simulink model "aie_hls"  (R2025a)
settings: Solver=VariableStepAuto  StartTime=0.0  StopTime=500  RelTol=1e-3
InitFcn:
  | %xmcCheckSlxPath(bdroot);
  | input = readcomplexdata('./sw/input.h');
undefined symbols (not defined in the file): S, Symmetric, vsva2197, xcvc1902
libraries: aieUtilities x2, aieDSP x1, aieBasic x1, hlsBasic x1, simulink x1, vmcUtilities x1, dspsrcs4 x1
settings Model: Creator=abehbood  LastModifiedBy=robg
settings SolverCC: AlgebraicLoopSolver=TrustRegion
settings DebuggingCC: UnconnectedInputMsg=warning  UnconnectedOutputMsg=warning  UnconnectedLineMsg=warning
settings ModelReferenceCC: EnableRefExpFcnMdlSchedulingChecks=on
settings SFSimCC: CustomCodeUndefinedFunction=UseInterfaceOnly
settings RTWCC: GPUComputeCapability=3.5  DLArmComputeVersion=19.05

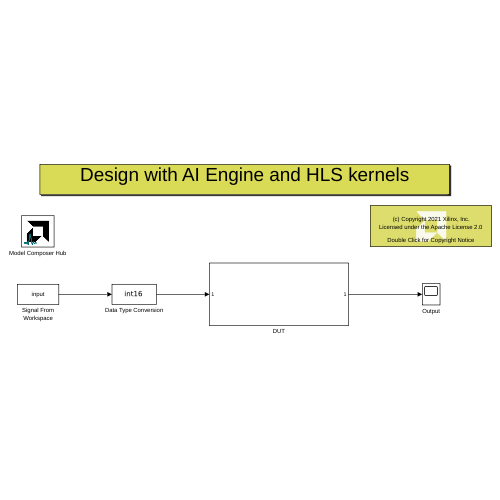
[thumbnail: Simulink's stored preview of the top-level diagram]
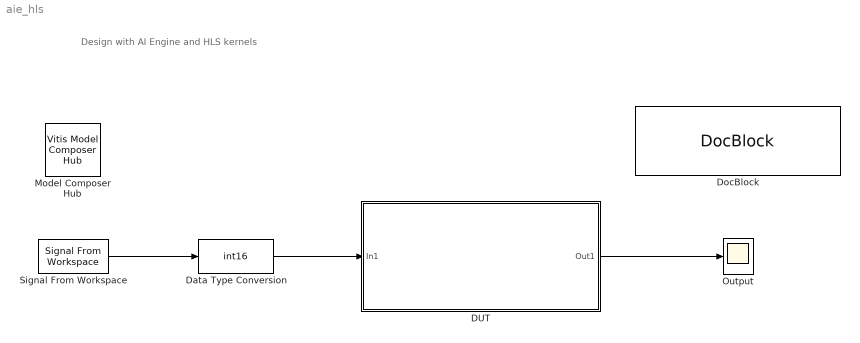
== system aie_hls ==
  note: Design with AI Engine and HLS kernels
  DUT : Subsystem
  Data Type Conversion : DataTypeConversion  OutDataTypeStr=int16  SaturateOnIntegerOverflow=off  RndMeth=Floor
  DocBlock : simulink/Model-Wide Utilities/DocBlock  DocumentType=Text  mask(DocBlock){}
      content=|
      | ///////////////////////////////////////////////////////////////////////////
      | // Copyright 2021 Xilinx
      | //
      | // Licensed under the Apache License, Version 2.0 (the "License");
      | // you may not use this file except in compliance with the License.
      | // You may obtain a copy of the License at
      | //
      | // http://www.apache.org/licenses/LICENSE-2.0
      | //
      | // Unless required by applicable law or agreed to in writing, software
      | // distributed under the License is distributed on an "AS IS" BASIS,
      | // WITHOUT WARRANTIES OR CONDITIONS OF ANY KIND, either express or implied.
      | // See the License for the specific language governing permissions and
      | // limitations under the License.
      | ///////////////////////////////////////////////////////////////////////////
      mask Display:
      | xmcDrawBlockIcon();
      | disp(['{\fontsize{10pt}(c) Copyright 2021' ' Xilinx, Inc.}\newline \newline '],'texmode','on');
      | disp('{\fontsize{10pt}Licensed under the Apache License 2.0}','texmode','on');
      | disp('\newline \newline \newline{\fontsize{10pt}Double Click for Copyright Notice}','texmode','on');
  Model Composer Hub : vmcUtilities/Vitis Model Composer Hub  Tag=genX  CodeGeneration=off  SubsystemName=DUT  BlockHierPath=aie_hls/DUT  CompilationType=VitisCompilation  SubsystemType=DUTNode  AIEArrayConfig=Use entire AIE array  StartColumn=1  NumberOfColumns=1  TargetDirectory=./code  exportDesign=on  analyzeDesign=off  validateDesignOnHw=off  ExportType=Vitis Subsystem  IpVendor=xilinx.com  IpLibrary=hls  IpVersion=1.0  IpHWLanguage=Verilog  AieCompilerOptions={}  AieSimulatorOptions={}  CreateTestbench=off  TestbenchStackSize=10  RunRtlSim=off  RunCSim=off  RunAieSim=on  enableSimulationTimeout=on  enableGraphIterations=on  AieSimTimeout=50000  AieGraphIterations=-1  RunAieSimProfiling=off  LaunchVitisAnalyzer=off  PlotOutput=off  RunX86Sim=off  X86SimTimeout=10  GenHwImage=off  GenLibadfXo=on  GenHwValidationCode=on  PlatformType=Not Specified  HwSystemType=Baremetal  HwValidationTarget=hw  ProjDevice=xcvc1902-vsva2197-1LP-e-S  ProjDevicePart=xcvc1902-vsva2197-1LP-e-S  AIEType=AIE  SamplePeriod=-1  ClockFrequency=200  DataPathParallelism=1  xilinxfamily=versalaicore  part=xcvc1902  speed=-1LP-e-S  package=vsva2197  directory=./netlist  testbench=off  incr_netlist=off  synthesis_tool=Vivado  clock_wrapper=Clock Enables  dbl_ovrd=According to Block Masks  dcm_input_clock_period=10  sysclk_period=10  simulink_period=1  eval_field=0  IPInfoJsonString="{\"DUTSubsystemName\":\"DUT\",\"HLSKernel\":{\"SubsystemName\":\"polar_clip1\",\"FpgaClockFreq\":\"200\",\"IPName\":\"polar_clip1\",\"IPLibrary\":\"hls\",\"TargetDirectory\":\"./code\",\"FreqHz\":\"200000000\",\"KernelFunction\":\"polar_clip\"},\"SubsystemTag\":\"DUTNode\",\"AIESubsystem\":{\"SubsystemName\":\"AI_Engine1\",\"TargetDirectory\":\"./code\",\"AIEArrayConfig\":\"Use entire AIE array\",\"StartColumn\":\"1\",\"NumberOfColumns\":\"1\"}}"  LogFileName=/proj/xhdhdstaff5/sdegala/Head1/HEAD/ModelComposer_DEC_2025/Examples/AIENGINE_plus_PL/AIE_HLS/AIE_HLS_with_interface/code/model_composer.log  NThreads=4  IPConfigFile=/tmp/vmctmp-266926556510304559/aie_hls_ipconfig.json
  Output : Scope
      settings: ActiveDisplayYMinimum=-0.375  ActiveDisplayYMaximum=3.375
  Signal From Workspace : dspsrcs4/Signal From Workspace  X=input  Ts=(1/1e3)*128  nsamps=128  OutputAfterFinalValue=Setting to zero  ignoreOrWarnInputAndFrameLengths=off  OutputFrames=off
  wires:
  Data Type Conversion/1 -> DUT/1(In1)
  DUT/1(Out1) -> Output/1
  Signal From Workspace/1 -> Data Type Conversion/1

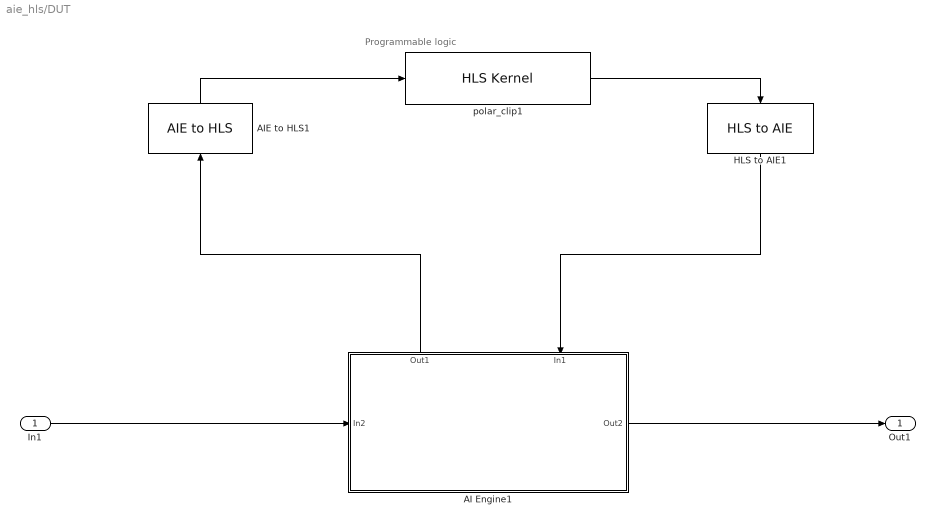
== system aie_hls/DUT ==
  note: Programmable logic
  In1 : Inport
  AI Engine1 : Subsystem
      settings: PortSchema="{\"entries\":[{\"content\":{\"sides\":[{\"content\":{\"connectorIds\":[\"In1\"]},\"type\":\"ConnectorPlacement.EquallySpacedRectSide\",\"uuid\":\"4c582470-6e07-4cf2-89ba-1d9148c6c342\"},{\"content\":{\"connectorIds\":[\"Out1\"],\"side\":\"RIGHT\"},\"type\":\"ConnectorPlacement.EquallySpacedRectSide\",\"uuid\":\"202127b6-913d-45d6-97d3-63d531af815e\"},{\"content\":{\"connectorIds\":[\"Out2\",\"In2\"],\"side\":\"TOP\"},\"type\":\"ConnectorPlacement.EquallySpacedRectSide\",\"uuid\":\"5b5cfc98-70f5-4b9e-bee7-2ee5eb3017f9\"}]},\"type\":\"ConnectorPlacement.EquallySpacedConnector\",\"uuid\":\"3aebc8b4-6a22-4c89-86c8-92d2be0437af\"}],\"packageUris\":[\"http://schema.mathworks.com/mf0/Connector/R2020b\"],\"version\":\"1.0\"}"
  AIE to HLS1 : aieUtilities/AIE to HLS  OutputType=int32  OutputSize=64  AllowMultiRate=on  InputType=cint16
  HLS to AIE1 : aieUtilities/HLS to AIE  OutputType=cint16  OutputSize=128  AllowMultiRate=on  InputType=int32
  polar_clip1 : hlsBasic/HLS Kernel  PortNames={}  PortSerializedTypes={}  FunctionTemplateParamNames={}  FunctionTemplateParamKinds={}  FunctionTemplateParamTypes={}  FunctionTemplateParamValues={}  PortSynchronicities={'auto'; 'auto'}  PortSignalSizes={0.000000000000000000e+00; 6.400000000000000000e+01}  PortParameterValues={}  PortAttributesTable={ 'Input', 'in_sample', 'hls::stream< hls::axis< ap_int< 32 >, 0, 0, 0 >, 0 > &', '', ''; 'Output', 'out_sample', 'hls::stream< hls::axis< ap_int< 32 >, 0, 0, 0 >, 0 > &', '', '64' }  PortAttributesEnablement={'off', 'off', 'off', 'off', 'off';'off', 'off', 'off', 'off', 'on'}  PortParametersTable={}  SampleTime=-1  PortDirectionTable={ 'in_sample', 'hls::stream< hls::axis< ap_int< 32 >, 0, 0, 0 >, 0 > &', 'Input', 'Port'; 'out_sample', 'hls::stream< hls::axis< ap_int< 32 >, 0, 0, 0 >, 0 > &', 'Output', 'Port' }  FunctionTemplateParams={}  FunctionTemplateParamsEnables={}  FunctionTemplateParamsVisible=off  FunctionDeclTypeOptions=C[1 1]@t7@<empty>  PortDirectionTabVisible=on  ArgDirections={1.000000000000000000e+00; 2.000000000000000000e+00}  ArgInterfaceTypes={}  FunctionIndex=1  FormalArgDecls={'hls::stream< hls::axis< ap_int< 32 >, 0, 0, 0 >, 0 > & in_sample', 'hls::stream< hls::axis< ap_int< 32 >, 0, 0, 0 >, 0 > & out_sample'}  SimLibPath=''  FunctionTabVisible=on  FunctionDescription=void polar_clip(hls::stream< hls::axis< ap_int< 32 >, 0, 0, 0 >, 0 > & in_sample, hls::stream< hls::axis< ap_int< 32 >, 0, 0, 0 >, 0 > & out_sample)  blockJsonConstraints=[]  deprecateConstraints=0  KernelHeaderFile=src/hls_kernels.h  KernelFunction=polar_clip  KernelFunctionSelect=<empty>  KernelSourceFile=src/polar_clip.cpp  KernelSearchPaths={}  PreProcOptions={}
  Out1 : Outport
  wires:
  HLS to AIE1/1 -> AI Engine1/2(In1)
  AIE to HLS1/1 -> polar_clip1/1
  AI Engine1/2(Out1) -> AIE to HLS1/1
  In1/1 -> AI Engine1/1(In2)
  polar_clip1/1 -> HLS to AIE1/1
  AI Engine1/1(Out2) -> Out1/1

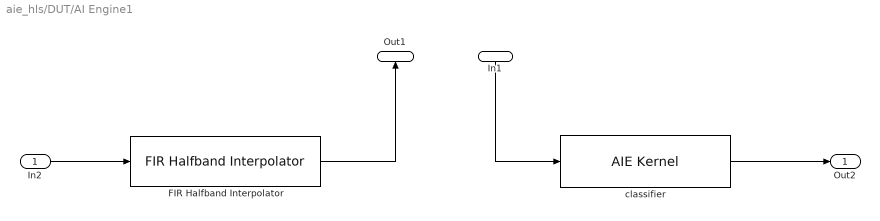
== system aie_hls/DUT/AI Engine1 ==
  In2 : Inport
  In1 : Inport  Port=2
  FIR Halfband Interpolator : aieDSP/FIR Halfband Interpolator  data_type=cint16  coef_type=int16  use_coeff_reload=off  dual_ip=off  num_outputs=off  coeff=[33, -158,491, -1214, 2674, -5942, 20503, 32767]  fir_length=31  input_window_size=128  shift_val=0  rnd_mode=Floor  sat_mode=3-Symmetric  interp_poly=1  upshift_ct=off  casc_length=1  AIE_VARIANT=1  TP_API=0  ssr=1  blockJsonConstraints=[]  blockJsonConstraintsInternal=[]  spec=vmc_fir_interpolate_hb.json  SerializedMaskParamNames=[]  SerializedMaskParamValues=[]  SerializedMaskParamVisibilities=[]  block_type=FIR Halfband Interpolator  SerializedMaskParamDataypes=typename|typename|uint|uint|uint|coef_type|uint|uint|uint|uint|uint|uint|uint|uint|uint|uint|uint  SerializedMaskParamEnumStrArr=0|0|0|0|0|0|0|0|0|Floor,Ceiling,Round to positive infinity,Round to negative infinity,Round symmetrical to infinity,Round symmetrical to zero,Round convergent to even,Round convergent to odd|0-None,1-Asymmetric,3-Symmetric|0|0|0|0|0|0  SerializedMaskParamEnumValArr=0|0|0|0|0|0|0|0|0|0,1,2,3,4,5,6,7|0,1,3|0|0|0|0|0|0  SerializedMaskParamVectorArr=0|0|0|0|0|1|0|0|0|0|0|0|0|0|0|0|0  SerializedMaskParamKeys=TT_DATA|TT_COEFF|TP_USE_COEFF_RELOAD|TP_DUAL_IP|TP_NUM_OUTPUTS|coeff|TP_FIR_LEN|TP_INPUT_WINDOW_VSIZE|TP_SHIFT|TP_RND|TP_SAT|TP_PARA_INTERP_POLY|TP_UPSHIFT_CT|TP_CASC_LEN|AIE_VARIANT|TP_API|TP_SSR
  classifier : aieBasic/AIE Kernel  KernelAllAttrs=s[12;12;9;9;19;14;21;23;24;21;12;24;26;26;26;27;28;9;21;23;23;23;24;25;14;19;19;29]@FunctionNameDeclFileNamePortNamesPortTypesPortSerializedTypesPortDirectionsPortWindowSizeEnablesPortWindowMarginEnablesPortSynchronicityEnablesPortSignalSizeEnablesFunctionDeclFunctionTemplateSpecKindFunctionTemplateParamNamesFunctionTemplateParamKindsFunctionTemplateParamTypesFunctionTemplateParamValuesFunctionTemplateParamEnablesClassDeclClassTemplateSpecKindClassTemplateParamNamesClassTemplateParamKindsClassTemplateParamTypesClassTemplateParamValuesClassTemplateParamEnablesClassCtorDeclsClassCtorParamNamesClassCtorParamTypesClassCtorParamSerializedTypes[1 1]@C[28 1]@t10@classifiert19@../../src/kernels.hC[2 1]@t5@inputt6@outputC[2 1]@t21@input_stream_cint16 *t21@output_window_int32 *C[2 1]@t33@{P{Tinput_stream{1{t{Scint16}}}}}t31@{P{Toutput_window{1{t{Bi32}}}}}C[2 1]@t5@inputt6@outputC[2 1]@l0@l1@C[2 1]@l0@l0@C[2 1]@l0@l1@C[2 1]@l0@l0@t74@void classifier(input_stream_cint16 * input, output_window_int32 * output)t4@nonee[0 1]@e[0 1]@e[0 1]@e[0 1]@e[0 1]@nne[0 1]@e[0 1]@e[0 1]@e[0 1]@e[0 1]@e[0 1]@e[0 1]@e[0 1]@e[0 1]@  PortNames={'input'; 'output'}  PortSerializedTypes={'{P{Tinput_stream{1{t{Scint16}}}}}'; '{P{Toutput_window{1{t{Bi32}}}}}'}  PortWindowSizes={0.000000000000000000e+00, 1.280000000000000000e+02}  PortWindowMargins={0.000000000000000000e+00, 0.000000000000000000e+00}  PortSynchronicities={'auto', 'sync'}  PortSignalSizes={0.000000000000000000e+00; 0.000000000000000000e+00}  FunctionTemplateSpecKind=none  FunctionTemplateParamNames={}  FunctionTemplateParamKinds={}  FunctionTemplateParamTypes={}  FunctionTemplateParamValues={}  FunctionIndex=1  FunctionTabVisible=on  FunctionTemplateParamsVisible=off  FunctionDeclTypeOptions=C[1 1]@t74@void classifier(input_stream_cint16 * input, output_window_int32 * output)  FunctionDecl=void classifier(input_stream_cint16 * input, output_window_int32 * output)  FunctionTemplateParams={}  FunctionTemplateParamsEnables={}  PortAttrs={ 'Input', 'input', 'input_stream_cint16 *', '', '', '', ''; 'Output', 'output', 'output_window_int32 *', '128', '', 'sync', '' }  PortAttrsEnables={'off', 'off', 'off', 'off', 'off', 'off', 'off';'off', 'off', 'off', 'on', 'off', 'on', 'off'}  SampleTime=-1  KernelHeaderFile=src/kernels.h  KernelFunction=classifier  KernelSourceFile=src/kernels/classifiers/classify.cc  KernelSearchPaths={}  PreProcOptions={}  blockJsonConstraints=[]
  Out2 : Outport  VectorParamsAs1DForOutWhenUnconnected=off
  Out1 : Outport  Port=2  VectorParamsAs1DForOutWhenUnconnected=off
  wires:
  FIR Halfband Interpolator/1 -> Out1/1
  In2/1 -> FIR Halfband Interpolator/1
  In1/1 -> classifier/1
  classifier/1 -> Out2/1
